simulink model "optimized_airport_sim"  (R2021a)
settings: Solver=VariableStepAuto  StartTime=0.0  StopTime=1e5  RelTol=1e-3
undefined symbols (not defined in the file): m, n
settings Model: Creator=hagarusama  LastModifiedBy=hagarusama

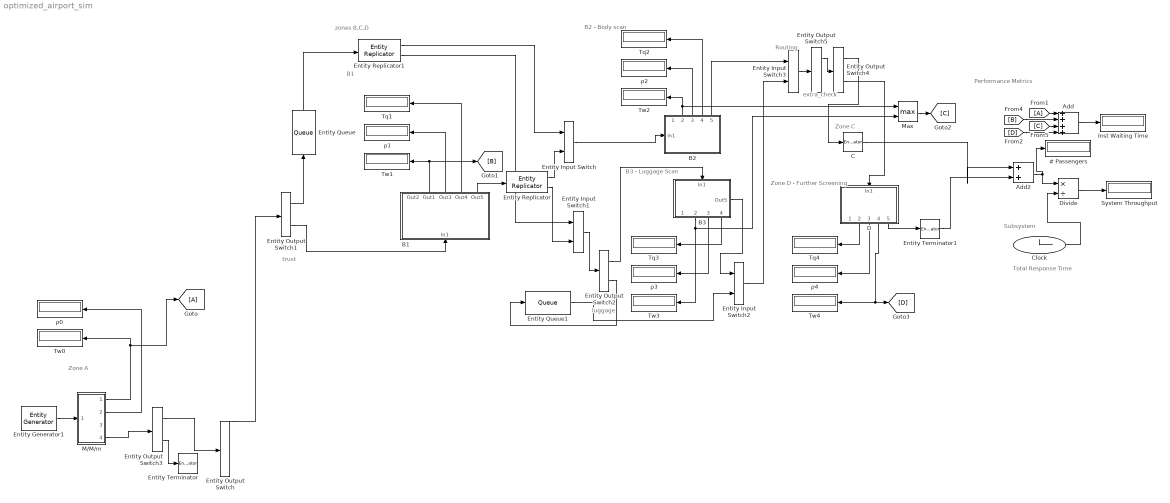
== system optimized_airport_sim ==
  note: trust
  note: B2 -
      | Body
      | scan
  note: zones B,C,D
  note: B3 -
      | Luggage
      | Scan
  note: Performance Metrics
  note: Zone D -
      |
      | Further
      | Screening
  note: B1
  note: Zone A
  note: Subsystem
  note: Zone C
  note: Total Response Time
  note: Routing
  note: luggage
  note: extra_check
  # Passengers : Display
  Add : Sum  Inputs=++++  SaturateOnIntegerOverflow=on
  Add2 : Sum
  B1 : Subsystem
  B2 : Subsystem
      settings: PortSchema="{\"entries\":[{\"content\":{\"sides\":[{\"content\":{\"connectorIds\":[]},\"type\":\"ConnectorPlacement.EquallySpacedRectSide\",\"uuid\":\"7ea955c4-59a0-4b16-a665-3c7419b36f79\"},{\"content\":{\"connectorIds\":[\"Out1\",\"Out2\",\"Out3\",\"Out4\",\"Out5\"],\"side\":\"RIGHT\"},\"type\":\"ConnectorPlacement.EquallySpacedRectSide\",\"uuid\":\"a8a3c229-e196-4360-bdfa-8ef645b2ce9c\"},{\"content\":{\"connectorIds\":[\"In1\"],\"side\":\"TOP\"},\"type\":\"ConnectorPlacement.EquallySpacedRectSide\",\"uuid\":\"5260f7b5-f6e8-463a-b0c5-598c56357d98\"}]},\"type\":\"ConnectorPlacement.EquallySpacedConnector\",\"uuid\":\"58c66fb9-1797-41d8-b8ed-62a065428871\"}],\"packageUris\":[\"http://schema.mathworks.com/mf0/Connector/R2020b\"],\"version\":\"1.0\"}"
  B3 : Subsystem
      settings: PortSchema="{\"entries\":[{\"content\":{\"sides\":[{\"content\":{\"connectorIds\":[\"In1\"]},\"type\":\"ConnectorPlacement.EquallySpacedRectSide\",\"uuid\":\"7ea955c4-59a0-4b16-a665-3c7419b36f79\"},{\"content\":{\"connectorIds\":[\"Out1\",\"Out2\",\"Out3\",\"Out4\"],\"side\":\"RIGHT\"},\"type\":\"ConnectorPlacement.EquallySpacedRectSide\",\"uuid\":\"a8a3c229-e196-4360-bdfa-8ef645b2ce9c\"},{\"content\":{\"connectorIds\":[],\"side\":\"TOP\"},\"type\":\"ConnectorPlacement.EquallySpacedRectSide\",\"uuid\":\"5260f7b5-f6e8-463a-b0c5-598c56357d98\"},{\"content\":{\"connectorIds\":[\"Out5\"],\"side\":\"BOTTOM\"},\"type\":\"ConnectorPlacement.EquallySpacedRectSide\",\"uuid\":\"b778f381-c9da-4203-8e39-7c353a561693\"}]},\"type\":\"ConnectorPlacement.EquallySpacedConnector\",\"uuid\":\"58c66fb9-1797-41d8-b8ed-62a065428871\"}],\"packageUris\":[\"http://schema.mathworks.com/mf0/Connector/R2020b\"],\"version\":\"1.0\"}"
  C : EntityTerminator  InputPortMessageModes=m  NumberEntitiesArrived=on
      settings: OutputPortMap=o0
  Clock : Clock
  D : Subsystem
  Divide : Product  Inputs=*/  SaturateOnIntegerOverflow=on
  Entity Input Switch : EntityInputSwitch  InputPortMessageModes=m,m  OutputPortMessageModes=m
  Entity Input Switch1 : EntityInputSwitch  InputPortMessageModes=m,m  OutputPortMessageModes=m
  Entity Input Switch2 : EntityInputSwitch  InputPortMessageModes=m,m  OutputPortMessageModes=m
  Entity Input Switch3 : EntityInputSwitch  InputPortMessageModes=m,m  OutputPortMessageModes=m  ActivePortSelection=Switch  SwitchingCriterion=Equiprobable  Seed=450279
  Entity Output Switch : EntityOutputSwitch  InputPortMessageModes=m  OutputPortMessageModes=m,m,m,m,m,m,m,m,m,m,m,m,m,m,m,m,m,m  NumberOutputPorts=18  SwitchingCriterion=Equiprobable  Seed=9647085  SwitchAttributeName=Attribute1
      settings: OutputPortMap=o0,o1,o2,o3,o4,o5,o6,o7,o8,o9,o10,o11,o12,o13,o14,o15,o16,o17
  Entity Output Switch1 : EntityOutputSwitch  InputPortMessageModes=m  OutputPortMessageModes=m,m  SwitchingCriterion=From attribute  Seed=9647085  SwitchAttributeName=trust
  Entity Output Switch2 : EntityOutputSwitch  InputPortMessageModes=m  OutputPortMessageModes=m,m  SwitchingCriterion=From attribute  SwitchAttributeName=luggage
  Entity Output Switch3 : EntityOutputSwitch  InputPortMessageModes=m  OutputPortMessageModes=m,m  SwitchingCriterion=From attribute  Seed=9647085  SwitchAttributeName=valid
  Entity Output Switch4 : EntityOutputSwitch  InputPortMessageModes=m  OutputPortMessageModes=m,m  SwitchingCriterion=From attribute  Seed=9632160  SwitchAttributeName=extra_check
  Entity Output Switch5 : EntityOutputSwitch  InputPortMessageModes=m  OutputPortMessageModes=m,m  SwitchingCriterion=Equiprobable  Seed=604377
  Entity Generator1 : EntityGenerator  OutputPortMessageModes=m  TimeSource=MATLAB action  IntergenerationTimeAction=|  GenerateAction=|  AttributeName=trust|luggage|valid|extra_check|rand  AttributeInitialValue=1|1|1|1|0.9  EntityType=Structured  EntityTypeName=Entity
      IntergenerationTimeAction=|
      | dt = rand(1,1);
      | persistent rngInit;
      | if isempty(rngInit)
      |     seed = 153503;
      |     rng(seed);
      |     rngInit = true;
      | end
      | 
      | % Pattern: Exponential distribution
      | mu = 0.5;
      | dt = -mu * log(1 - rand());
      GenerateAction=|
      | % entity.trust = 2;
      | % entity.luggage = 1;
      | 
      | entity.rand = rand();
      |   if 0.02 <= entity.rand
      |      entity.extra_check = 1;
      |   else
      |      entity.extra_check = 2;
      |   end
      | 
      |   if 0.55 <= entity.rand
      |      entity.trust = 1;
      |   else
      |      entity.trust = 2;
      |   end
      | 
      |   if 0.2 <= entity.rand
      |      entity.luggage = 1;
      |   else
      |     entity.luggage = 2;
      |   end
  Entity Queue : Queue  InputPortMessageModes=m  OutputPortMessageModes=m  Capacity=inf
  Entity Queue1 : Queue  InputPortMessageModes=m  OutputPortMessageModes=m  Capacity=Inf
  Entity Replicator : EntityReplicator  InputPortMessageModes=m  OutputPortMessageModes=m,m
  Entity Replicator1 : EntityReplicator  InputPortMessageModes=m  OutputPortMessageModes=m,m
  Entity Terminator : EntityTerminator  InputPortMessageModes=m
  Entity Terminator1 : EntityTerminator  InputPortMessageModes=m  NumberEntitiesArrived=on
      settings: OutputPortMap=o0
  Inst Waiting Time : Display
  M/M/m : Subsystem
  Max : MinMax  Function=max  Inputs=2
  System Throughput : Display
  Tq{1..4} (4 alike) : Display
  Tw{0..4} (5 alike) : Display
  ρ{0..4} (5 alike) : Display
  wires:
  B3/4(Out4) -> Tq3/1
  Entity Replicator1/2 -> Entity Input Switch1/1
  Clock/1 -> Divide/2
  Entity Replicator/2 -> Entity Input Switch1/2
  B2/2(Out1) -> Max/1, Tw2/1
  D/5(Out5) -> Entity Terminator1/1
  Entity Input Switch/1 -> B2/1(In1)
  Entity Queue/1 -> Entity Replicator1/1
  B1/5(Out5) -> Entity Replicator/1
  B1/3(Out3) -> ρ1/1
  M/M/m/4(Out4) -> Entity Output Switch3/1
  Entity Replicator/1 -> Entity Input Switch/2
  Entity Replicator1/1 -> Entity Input Switch/1
  Entity Output Switch4/1 -> C/1
  Entity Generator1/1 -> M/M/m/1(In1)
  Entity Output Switch4/2 -> D/1(In1)
  Entity Output Switch1/1 -> Entity Queue/1
  Entity Output Switch1/2 -> B1/1(In1)
  B1/2(Out1) -> Tw1/1, [B]
  B3/2(Out1) -> Tw3/1, Max/2
  Add/1 -> Inst Waiting Time/1
  B2/3(Out3) -> ρ2/1
  D/4(Out4) -> Tw4/1, [D]
  B3/3(Out3) -> ρ3/1
  Add2/1 -> # Passengers/1, Divide/1
  C/1 -> Add2/1
  Divide/1 -> System Throughput/1
  Entity Output Switch/1 -> Entity Output Switch1/1
  D/3(Out3) -> ρ4/1
  B1/4(Out4) -> Tq1/1
  D/2(Out1) -> Tq4/1
  B2/4(Out4) -> Tq2/1
  Entity Output Switch2/2 -> Entity Queue1/1
  Entity Input Switch1/1 -> Entity Output Switch2/1
  Entity Output Switch2/1 -> B3/1(In1)
  B3/5(Out5) -> Entity Input Switch2/1
  Entity Queue1/1 -> Entity Input Switch2/2
  Entity Input Switch2/1 -> Entity Input Switch3/2
  M/M/m/1(Out1) -> [A], Tw0/1
  M/M/m/2(Out2) -> ρ0/1
  Entity Output Switch3/1 -> Entity Output Switch/1
  Entity Output Switch3/2 -> Entity Terminator/1
  Entity Output Switch5/1 -> Entity Output Switch4/1
  Entity Input Switch3/1 -> Entity Output Switch5/1
  B2/5(Out5) -> Entity Input Switch3/1
  Entity Terminator1/1 -> Add2/2
  Max/1 -> [C]
  [A] -> Add/1
  [B] -> Add/2
  [C] -> Add/3
  [D] -> Add/4

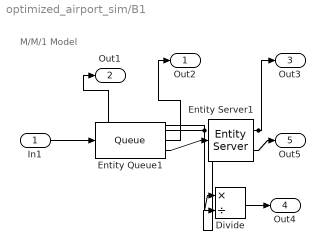
== system optimized_airport_sim/B1 ==
  note: M/M/1 Model
  In1 : Inport
  Divide : Product  Inputs=*/
  Entity Queue1 : Queue  InputPortMessageModes=m  OutputPortMessageModes=n,n,m  Capacity=inf  AverageWait=on  AverageQueueLength=on
      settings: OutputPortMap=o2,o3,o5
  Entity Server1 : EntityServer  InputPortMessageModes=m  OutputPortMessageModes=n,m  Capacity=1  ServiceTimeSource=MATLAB action  ServiceTimeAction=|  Utilization=on
      | dt = rand(1,1);
      | persistent rngInit;
      | if isempty(rngInit)
      |     seed = 2273520;
      |     rng(seed);
      |     rngInit = true;
      | end
      | 
      | % Pattern: Exponential distribution
      | mu = 15;
      | dt = -mu * log(1 - rand());
      settings: OutputPortMap=o5,o9
  Out2 : Outport
  Out1 : Outport  Port=2
  Out3 : Outport  Port=3
  Out4 : Outport  Port=4
  Out5 : Outport  Port=5
  wires:
  In1/1 -> Entity Queue1/1
  Entity Queue1/2 -> Out2/1
  Entity Server1/1 -> Divide/2, Out3/1
  Entity Queue1/1 -> Divide/1, Out1/1
  Entity Queue1/3 -> Entity Server1/1
  Entity Server1/2 -> Out5/1
  Divide/1 -> Out4/1

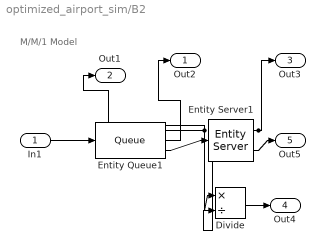
== system optimized_airport_sim/B2 ==
  note: M/M/1 Model
  In1 : Inport
  Divide : Product  Inputs=*/
  Entity Queue1 : Queue  InputPortMessageModes=m  OutputPortMessageModes=n,n,m  Capacity=inf  AverageWait=on  AverageQueueLength=on
      settings: OutputPortMap=o2,o3,o5
  Entity Server1 : EntityServer  InputPortMessageModes=m  OutputPortMessageModes=n,m  Capacity=1  ServiceTimeSource=MATLAB action  ServiceTimeAction=|  Utilization=on
      | dt = rand(1,1);
      | persistent rngInit;
      | if isempty(rngInit)
      |     seed = 7612432;
      |     rng(seed);
      |     rngInit = true;
      | end
      | 
      | % Pattern: Exponential distribution
      | mu = 7;
      | dt = -mu * log(1 - rand());
      settings: OutputPortMap=o5,o9
  Out2 : Outport
  Out1 : Outport  Port=2
  Out3 : Outport  Port=3
  Out4 : Outport  Port=4
  Out5 : Outport  Port=5
  wires:
  Divide/1 -> Out4/1
  Entity Server1/2 -> Out5/1
  Entity Queue1/3 -> Entity Server1/1
  Entity Queue1/1 -> Out1/1, Divide/1
  Entity Server1/1 -> Out3/1, Divide/2
  Entity Queue1/2 -> Out2/1
  In1/1 -> Entity Queue1/1

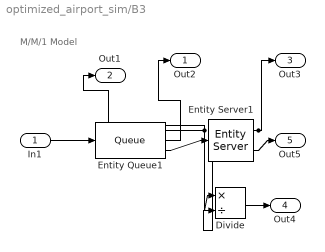
== system optimized_airport_sim/B3 ==
  note: M/M/1 Model
  In1 : Inport
  Divide : Product  Inputs=*/
  Entity Queue1 : Queue  InputPortMessageModes=m  OutputPortMessageModes=n,n,m  Capacity=inf  AverageWait=on  AverageQueueLength=on
      settings: OutputPortMap=o2,o3,o5
  Entity Server1 : EntityServer  InputPortMessageModes=m  OutputPortMessageModes=n,m  Capacity=1  ServiceTimeSource=MATLAB action  ServiceTimeAction=|  Utilization=on
      | dt = rand(1,1);
      | persistent rngInit;
      | if isempty(rngInit)
      |     seed = 6069205;
      |     rng(seed);
      |     rngInit = true;
      | end
      | 
      | % Pattern: Exponential distribution
      | mu = 8;
      | dt = -mu * log(1 - rand());
      settings: OutputPortMap=o5,o9
  Out2 : Outport
  Out1 : Outport  Port=2
  Out3 : Outport  Port=3
  Out4 : Outport  Port=4
  Out5 : Outport  Port=5
  wires:
  In1/1 -> Entity Queue1/1
  Entity Queue1/2 -> Out2/1
  Entity Server1/1 -> Divide/2, Out3/1
  Entity Queue1/1 -> Divide/1, Out1/1
  Entity Queue1/3 -> Entity Server1/1
  Entity Server1/2 -> Out5/1
  Divide/1 -> Out4/1

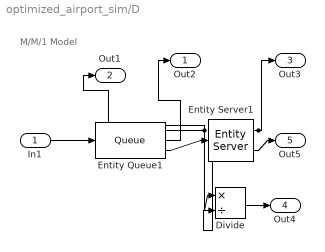
== system optimized_airport_sim/D ==
  note: M/M/1 Model
  In1 : Inport
  Divide : Product  Inputs=*/
  Entity Queue1 : Queue  InputPortMessageModes=m  OutputPortMessageModes=n,n,m  Capacity=inf  AverageWait=on  AverageQueueLength=on
      settings: OutputPortMap=o2,o3,o5
  Entity Server1 : EntityServer  InputPortMessageModes=m  OutputPortMessageModes=n,m  Capacity=1  ServiceTimeSource=MATLAB action  ServiceTimeAction=|  Utilization=on
      | dt = rand(1,1);
      | persistent rngInit;
      | if isempty(rngInit)
      |     seed = 6069205;
      |     rng(seed);
      |     rngInit = true;
      | end
      | 
      | % Pattern: Exponential distribution
      | mu = 60*3;
      | dt = -mu * log(1 - rand());
      settings: OutputPortMap=o5,o9
  Out2 : Outport
  Out1 : Outport  Port=2
  Out3 : Outport  Port=3
  Out4 : Outport  Port=4
  Out5 : Outport  Port=5
  wires:
  Divide/1 -> Out4/1
  Entity Server1/2 -> Out5/1
  Entity Queue1/3 -> Entity Server1/1
  Entity Queue1/1 -> Out1/1, Divide/1
  Entity Server1/1 -> Out3/1, Divide/2
  Entity Queue1/2 -> Out2/1
  In1/1 -> Entity Queue1/1

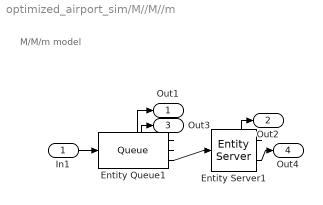
== system optimized_airport_sim/M//M//m ==
  note: M/M/m model
  In1 : Inport
  Entity Queue1 : Queue  InputPortMessageModes=m  OutputPortMessageModes=n,n,m  Capacity=inf  AverageWait=on  AverageQueueLength=on
      settings: OutputPortMap=o2,o3,o5
  Entity Server1 : EntityServer  InputPortMessageModes=m  OutputPortMessageModes=n,m  Capacity=18  ServiceTimeSource=MATLAB action  ServiceTimeAction=|  ServiceCompleteAction=|  Utilization=on
      ServiceTimeAction=|
      | dt = rand(1,1);
      | persistent rngInit;
      | if isempty(rngInit)
      |     seed = 8084213;
      |     rng(seed);
      |     rngInit = true;
      | end
      | 
      | % Pattern: Exponential distribution
      | mu = 5;
      | dt = -mu * log(1 - rand());
      ServiceCompleteAction=|
      | if 0.15 <= rand()
      |   entity.valid = 1;
      | else
      |   entity.valid =2;
      | end
      settings: OutputPortMap=o5,o9
  Out1 : Outport
  Out2 : Outport  Port=2
  Out3 : Outport  Port=3
  Out4 : Outport  Port=4
  wires:
  Entity Queue1/3 -> Entity Server1/1
  Entity Queue1/1 -> Out3/1
  In1/1 -> Entity Queue1/1
  Entity Queue1/2 -> Out1/1
  Entity Server1/2 -> Out4/1
  Entity Server1/1 -> Out2/1
